simulink model "Torque_Vectoring_2RWD"  (R2023a)
settings: Solver=VariableStepAuto  StartTime=0.0  StopTime=10.0  RelTol=1e-3
undefined symbols (not defined in the file): Treq
libraries: slpidlib x1
settings Model: Creator=MOHAMED IBRAHIM  LastModifiedBy=M3tal
settings SolverCC: AlgebraicLoopSolver=TrustRegion

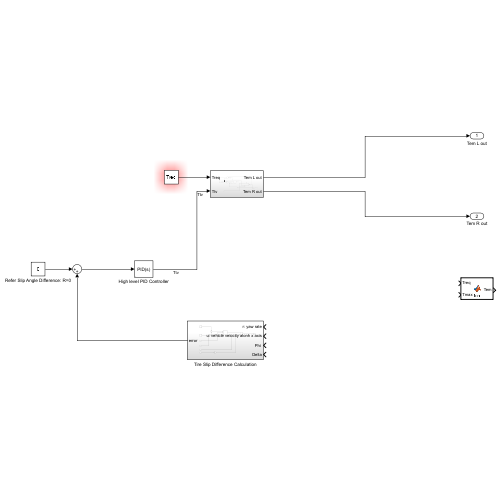
[thumbnail: Simulink's stored preview of the top-level diagram]
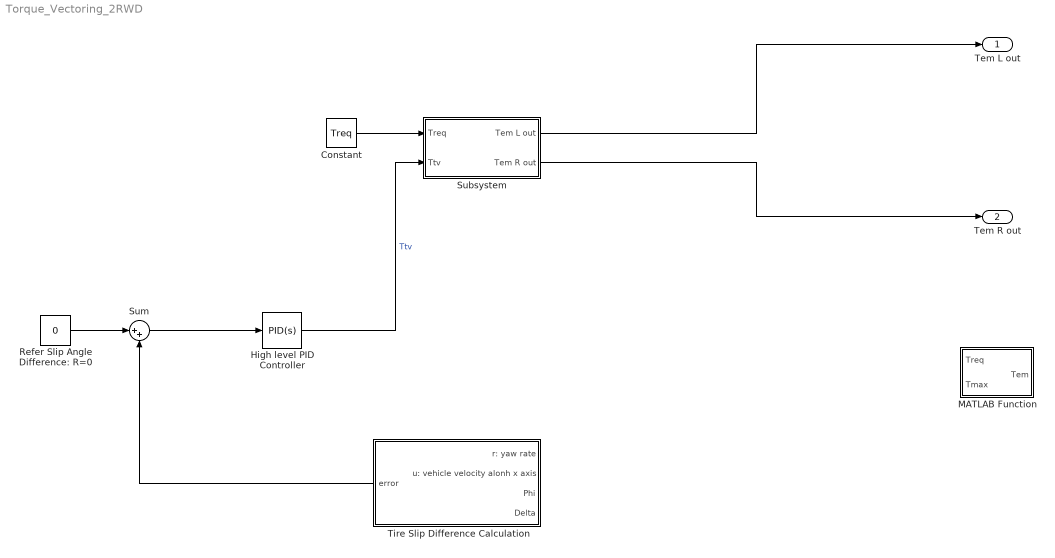
== system Torque_Vectoring_2RWD ==
  Constant : Constant  Value=Treq
  High level PID Controller : slpidlib/PID Controller  Controller=PID  Form=Parallel  TimeDomain=Continuous-time  UseExternalTs=off  SampleTime=-1  IntegratorMethod=Forward Euler  FilterMethod=Forward Euler  ControllerParametersSource=internal  P=1  I=1  UseKiTs=off  D=0  N=100  UseFilter=on  TunerSelectOption=Transfer Function Based (PID Tuner App)  InitialConditionSource=internal  InitialConditionForIntegrator=0  InitialConditionForFilter=0  DifferentiatorICPrevScaledInput=0  ExternalReset=none  TrackingMode=off  Kt=1  LimitOutput=off  SatLimitsSource=internal  UpperSaturationLimit=inf  LowerSaturationLimit=-inf  LinearizeAsGain=on  AntiWindupMode=none  Kb=1  LimitIntegrator=off  UpperIntegratorSaturationLimit=inf  LowerIntegratorSaturationLimit=-inf  POutMin=[]  POutMax=[]  IOutMin=[]  IOutMax=[]  DOutMin=[]  DOutMax=[]  NOutMin=[]  NOutMax=[]  SumOutMin=[]  SumOutMax=[]  SaturationOutMin=[]  SaturationOutMax=[]  PParamMin=[]  PParamMax=[]  IParamMin=[]  IParamMax=[]  DParamMin=[]  DParamMax=[]  NParamMin=[]  NParamMax=[]  KbParamMin=[]  KbParamMax=[]  KtParamMin=[]  KtParamMax=[]  KbOutMin=[]  KbOutMax=[]  KtOutMin=[]  KtOutMax=[]  IntegratorOutMin=[]  IntegratorOutMax=[]  FilterOutMin=[]  FilterOutMax=[]  SumI1OutMin=[]  SumI1OutMax=[]  SumI2OutMin=[]  SumI2OutMax=[]  SumI3OutMin=[]  SumI3OutMax=[]  SumI4OutMin=[]  SumI4OutMax=[]  SumDOutMin=[]  SumDOutMax=[]  DifferentiatorOutMin=[]  DifferentiatorOutMax=[]  FilterDiffOutCoefMin=[]  FilterDiffOutCoefMax=[]  ReciprocalOutMin=[]  ReciprocalOutMax=[]  SumDenOutMin=[]  SumDenOutMax=[]  SumNumOutMin=[]  SumNumOutMax=[]  DivideOutMin=[]  DivideOutMax=[]  UdiffTsProdOutMin=[]  UdiffTsProdOutMax=[]  NTsProdOutMin=[]  NTsProdOutMax=[]  UintegralTsProdOutMin=[]  UintegralTsProdOutMax=[]  UngainTsProdOutMin=[]  UngainTsProdOutMax=[]  ClampingZeroOutDataTypeStr=Inherit: Inherit via back propagation  ClampingZeroOutMin=[]  ClampingZeroOutMax=[]  FilterDenConstantOutDataTypeStr=Inherit: Inherit via back propagation  FilterDenConstantOutMin=[]  FilterDenConstantOutMax=[]  PCopyOutDataTypeStr=Inherit: Inherit via back propagation  PCopyOutMin=[]  PCopyOutMax=[]  NCopyOutDataTypeStr=Inherit: Inherit via back propagation  NCopyOutMin=[]  NCopyOutMax=[]  IntegratorContinuousStateAttributes=''  IntegratorStateMustResolveToSignalObject=off  IntegratorRTWStateStorageClass=Auto  FilterContinuousStateAttributes=''  FilterStateMustResolveToSignalObject=off  FilterRTWStateStorageClass=Auto  ParallelPVariant=InternalParameters  IdealPVariant=Disabled  IVariant=InternalParameters  DVariant=InternalParameters  IntegratorVariant=Continuous  SatVariant=Disabled  AWVariant=Passthrough  PCopyVariant=Disabled  TRVariant=Disabled  FdbkBlocksVariant=Forward  IdealPFdbkVariant=Disabled  SatFdbkVariant=Disabled  DerivativeFilterVariant=ContFilter  NVariant=InternalParameters  NCopyVariant=Disabled  FilterICVariant=InternalICsFilter  IntegratorICVariant=InternalICs  ExternalResetVariant=Disabled  TRSumVariant=Passthrough  SumFdbkVariant=Disabled  SumVariant=Sum_PID  TsampFilterVariant=InternalTs  TsampNgainVariant=Passthrough  TsampIntegralVariant=Disabled_SignalSpec  ExternalSaturationOutDataTypeStr=Inherit: Same as second input
  MATLAB Function : MATLAB Function  TreatAsAtomicUnit=on
  Refer Slip Angle Difference: R=0 : Constant  Value=0
  Subsystem : Subsystem
  Sum : Sum  Inputs=|++
  Tire Slip Difference Calculation : Subsystem
  Tem L out : Outport
  Tem R out : Outport  Port=2
  wires:
  Tire Slip Difference Calculation/1(error) -> Sum/2
  Refer Slip Angle Difference: R=0/1 -> Sum/1
  Sum/1 -> High level PID Controller/1
  High level PID Controller/1 -> Subsystem/2(Ttv)  "Ttv"
  Subsystem/1(Tem L out) -> Tem L out/1
  Subsystem/2(Tem R out) -> Tem R out/1
  Constant/1 -> Subsystem/1(Treq)

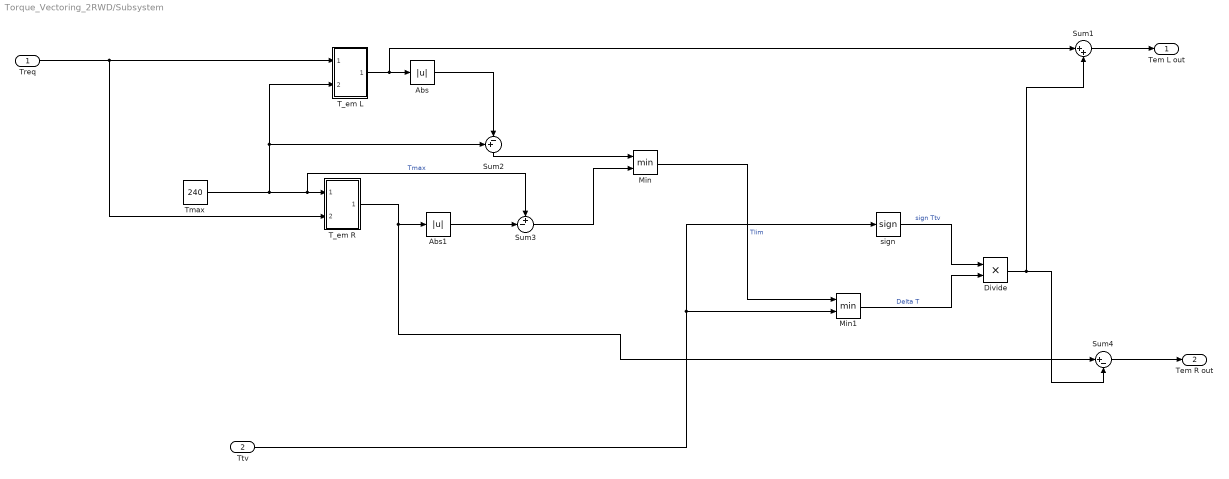
== system Torque_Vectoring_2RWD/Subsystem ==
  Treq : Inport
  Ttv : Inport  Port=2
  Abs : Abs  SaturateOnIntegerOverflow=off
  Abs1 : Abs  SaturateOnIntegerOverflow=off
  Divide : Product  Inputs=**
  Min : MinMax  Inputs=2
  Min1 : MinMax  Inputs=2
  Sum1 : Sum  Inputs=|++
  Sum2 : Sum  Inputs=+-|
  Sum3 : Sum  Inputs=+-|
  Sum4 : Sum  Inputs=|+-
  T_em L : Subsystem
  T_em R : Subsystem
  Tmax : Constant  Value=240
  sign : Signum
  Tem L out : Outport
  Tem R out : Outport  Port=2
  wires:
  Ttv/1 -> sign/1, Min1/2
  Abs1/1 -> Sum3/2
  Min/1 -> Min1/1  "Tlim"
  sign/1 -> Divide/1  "sign Ttv"
  Abs/1 -> Sum2/2
  T_em R/1(Output) -> Sum4/1, Abs1/1
  Tmax/1 -> Sum3/1, T_em R/1(Tmax), T_em L/2(Tmax), Sum2/1  "Tmax"
  Sum1/1 -> Tem L out/1
  Sum4/1 -> Tem R out/1
  T_em L/1(Output) -> Sum1/1, Abs/1
  Min1/1 -> Divide/2  "Delta T"
  Sum3/1 -> Min/2
  Sum2/1 -> Min/1
  Divide/1 -> Sum4/2, Sum1/2
  Treq/1 -> T_em R/2(Treq), T_em L/1(Treq)

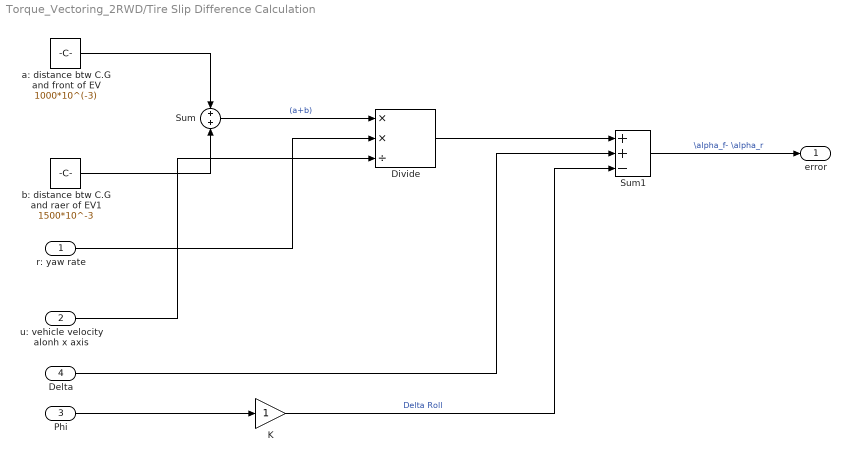
== system Torque_Vectoring_2RWD/Tire Slip Difference Calculation ==
  r: yaw rate : Inport
  u: vehicle velocity alonh x axis : Inport  Port=2
  "Phi " : Inport  Port=3
  Delta : Inport  Port=4
  Divide : Product  Inputs=**/
  K : Gain
  Sum : Sum  Inputs=+|+
  Sum1 : Sum  Inputs=+|+-
  a: distance btw C.G and front of EV : Constant  Value=1000*10^(-3)
  b: distance btw C.G and raer of EV1 : Constant  Value=1500*10^-3
  error : Outport
  wires:
  Delta/1 -> Sum1/2
  Sum/1 -> Divide/1  "(a+b)"
  Divide/1 -> Sum1/1
  u: vehicle velocity alonh x axis/1 -> Divide/3
  b: distance btw C.G and raer of EV1/1 -> Sum/2
  a: distance btw C.G and front of EV/1 -> Sum/1
  Sum1/1 -> error/1  "\\alpha_f- \\alpha_r"
  r: yaw rate/1 -> Divide/2
  "Phi "/1 -> K/1
  K/1 -> Sum1/3  "Delta Roll"

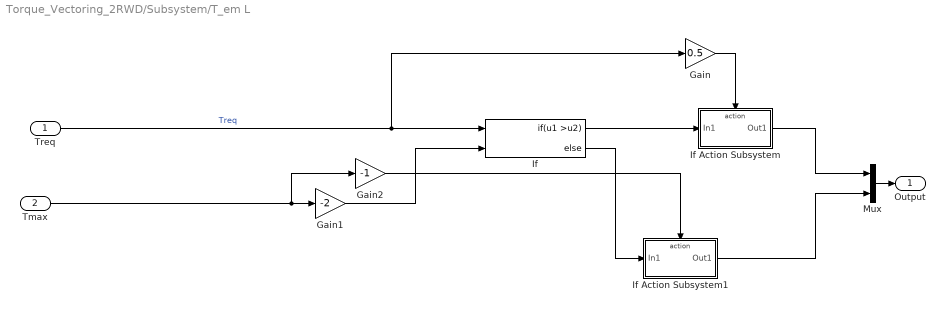
== system Torque_Vectoring_2RWD/Subsystem/T_em L ==
  Treq : Inport
  Tmax : Inport  Port=2
  Gain : Gain  Gain=0.5
  Gain1 : Gain  Gain=-2
  Gain2 : Gain  Gain=-1
  If : If  NumInputs=2  IfExpression=u1 >u2
  If Action Subsystem : Subsystem  TreatAsAtomicUnit=on
  If Action Subsystem1 : Subsystem  TreatAsAtomicUnit=on
  Mux : Mux  Inputs=2
  Output : Outport
  wires:
  Treq/1 -> Gain/1, If/1  "Treq"
  If Action Subsystem1/1(Out1) -> Mux/2
  Tmax/1 -> Gain2/1, Gain1/1
  Gain1/1 -> If/2
  Gain/1 -> If Action Subsystem/Action
  If/1 -> If Action Subsystem/1(In1)
  If/2 -> If Action Subsystem1/1(In1)
  If Action Subsystem/1(Out1) -> Mux/1
  Gain2/1 -> If Action Subsystem1/Action
  Mux/1 -> Output/1

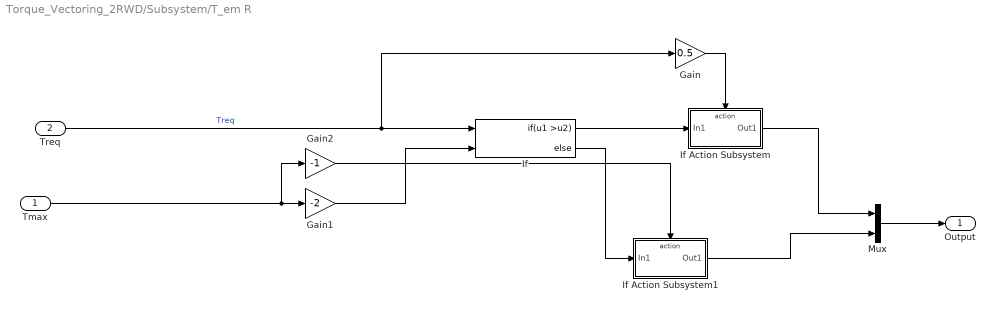
== system Torque_Vectoring_2RWD/Subsystem/T_em R ==
  Tmax : Inport
  Treq : Inport  Port=2
  Gain : Gain  Gain=0.5
  Gain1 : Gain  Gain=-2
  Gain2 : Gain  Gain=-1
  If : If  NumInputs=2  IfExpression=u1 >u2
  If Action Subsystem : Subsystem  TreatAsAtomicUnit=on
  If Action Subsystem1 : Subsystem  TreatAsAtomicUnit=on
  Mux : Mux  Inputs=2
  Output : Outport
  wires:
  Treq/1 -> Gain/1, If/1  "Treq"
  If Action Subsystem1/1(Out1) -> Mux/2
  Tmax/1 -> Gain2/1, Gain1/1
  Gain1/1 -> If/2
  Gain/1 -> If Action Subsystem/Action
  If/1 -> If Action Subsystem/1(In1)
  If/2 -> If Action Subsystem1/1(In1)
  If Action Subsystem/1(Out1) -> Mux/1
  Gain2/1 -> If Action Subsystem1/Action
  Mux/1 -> Output/1

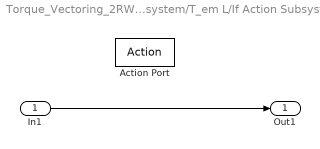
== system Torque_Vectoring_2RWD/Subsystem/T_em L/If Action Subsystem ==
  In1 : Inport
  Action Port : ActionPort
  Out1 : Outport
  wires:
  In1/1 -> Out1/1

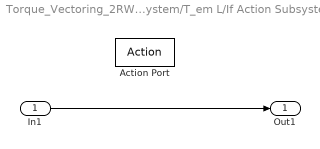
== system Torque_Vectoring_2RWD/Subsystem/T_em L/If Action Subsystem1 ==
  In1 : Inport
  Action Port : ActionPort
  Out1 : Outport
  wires:
  In1/1 -> Out1/1

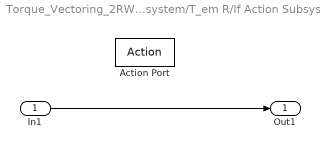
== system Torque_Vectoring_2RWD/Subsystem/T_em R/If Action Subsystem ==
  In1 : Inport
  Action Port : ActionPort
  Out1 : Outport
  wires:
  In1/1 -> Out1/1

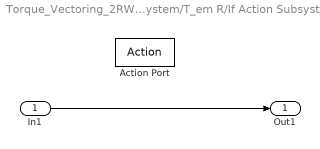
== system Torque_Vectoring_2RWD/Subsystem/T_em R/If Action Subsystem1 ==
  In1 : Inport
  Action Port : ActionPort
  Out1 : Outport
  wires:
  In1/1 -> Out1/1

== matlab function Torque_Vectoring_2RWD/MATLAB Function ==
  data: Treq input; Tem output; Tmax input
function Tem = fcn(Treq,Tmax)
if Treq > -2*Tmax
    Tem=Treq/2;
    else
    Tem=-Tmax;
    
end 
end
